simulink model "untitled"  (R2022a)
settings: Solver=VariableStepAuto  StartTime=0.0  StopTime=10.0  RelTol=1e-3
settings Model: Creator=12623  LastModifiedBy=12623

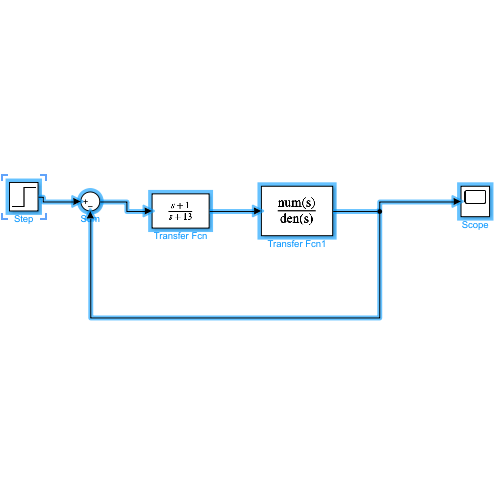
[thumbnail: Simulink's stored preview of the top-level diagram]
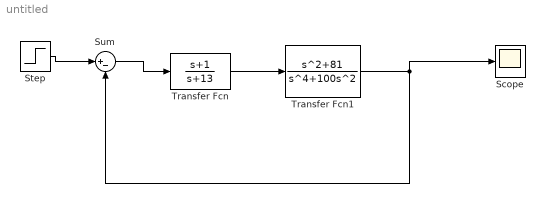
== system untitled ==
  Scope : Scope
  Step : Step  SampleTime=0
  Sum : Sum  Inputs=|+-
  Transfer Fcn : TransferFcn  Numerator=[1 1]  Denominator=[1 13]
  Transfer Fcn1 : TransferFcn  Numerator=[1 0 81]  Denominator=[1 0 100 0 0]
  wires:
  Sum/1 -> Transfer Fcn/1
  Transfer Fcn/1 -> Transfer Fcn1/1
  Transfer Fcn1/1 -> Scope/1, Sum/2
  Step/1 -> Sum/1
